simulink model "bike_model"  (R2018a)
settings: Solver=FixedStepAuto  StartTime=0.0  StopTime=10  FixedStep=Ts_IMU  RelTol=1e-3
values from neighbouring files (symbols this model uses):
  A_full = zeros(length(velocity_lqr),3,3)    [bike_init.m]
  A_full_dis = zeros(length(velocity_lqr),3,3)    [bike_init.m]
  amp_dist_roll_rate = 1    [bike_init.m]
  b = 1.095    [bike_init.m]    (also in bike_init_Merged_v1.m = bike3D190215())
  B_full = zeros(length(velocity_lqr),3)    [bike_init.m]
  B_full_dis = zeros(length(velocity_lqr),3)    [bike_init.m]
  C = eye(3)    [bike_init.m]    (also in bike_init_Merged_v1.m)
  complementary = 0.995    [bike_init.m]    (also in bike_init_Merged_v1.m = 0.985)
  cumulative_dist_along_path = [0;cumsum(dist_from_vertex_to_vertex,1)]    [bike_init.m]    (also in bike_init_Merged_v1.m)
  Dead_Band = [0.055,-0.005,0.005]    [bike_init.m]    (also in bike_init_Merged_v1.m = [0.055,-0.055,0.005])
  delay = 0.045    [bike_init.m]    (also in bike_init_Merged_v1.m)
  discrete = 1    [bike_init.m]
  dist_freq = 100    [bike_init.m]
  g = 9.81    [bike_init.m]    (also in bike_init_Merged_v1.m)
  IMU_height = 0.9    [bike_init.m]
  initial_x = x_ini_diff    (= 0)    [bike_init.m]    (also in bike_init_Merged_v1.m)
  initial_y = y_ini_diff    (= 0)    [bike_init.m]    (also in bike_init_Merged_v1.m)
  input_velocity = 2    [bike_init.m]    (also in bike_init_Merged_v1.m = 2.5)
  K_full = zeros(length(velocity_lqr),3)    [bike_init.m]
  K_full_dis = zeros(length(velocity_lqr),3)    [bike_init.m]    (also in bike_init_Merged_v1.m)
  L_full = zeros(length(velocity_lqr),3,3)    [bike_init.m]
  L_full_dis = zeros(length(velocity_lqr),3,3)    [bike_init.m]
  max_handlebar = 40*(pi/180)    (= 0.698131700798)    [bike_init.m]    (also in bike_init_Merged_v1.m)
  max_steering_motor_acc = inf    [bike_init.m]    (also in bike_init_Merged_v1.m)
  max_steering_motor_speed = 7.5    [bike_init.m]    (also in bike_init_Merged_v1.m)
  min_handlebar = -max_handlebar    (= -0.698131700798)    [bike_init.m]    (also in bike_init_Merged_v1.m)
  min_steering_motor_acc = -inf    [bike_init.m]    (also in bike_init_Merged_v1.m)
  min_steering_motor_speed = -7.5    [bike_init.m]    (also in bike_init_Merged_v1.m)
  noise_acc = 0.006*(pi/180)    (= 0.00010471975512)    [bike_init.m]    (also in bike_init_Merged_v1.m)
  noise_encoder = 1e-7    (= 1e-07)    [bike_init.m]    (also in bike_init_Merged_v1.m)
  noise_gyro = 0.001929307*(pi/180)    (= 3.36727594318e-05)    [bike_init.m]    (also in bike_init_Merged_v1.m)
  noise_hall = 0    [bike_init.m]    (also in bike_init_Merged_v1.m)
  parameters = [g h b a]    [bike_init.m]
  path_x = time_array    [bike_init.m]    (also in bike_init_Merged_v1.m)
  path_y = sqrt(path_x * 0.8) .* sin(0.1*path_x)    [bike_init.m]    (also in bike_init_Merged_v1.m)
  roll_rate_coef = 0.8    [bike_init.m]    (also in bike_init_Merged_v1.m = 0.9)
  Ts = 0.04    [bike_init.m]    (also in bike_init_Merged_v1.m)
  Ts_IMU = 0.01    [bike_init.m]    (also in bike_init_Merged_v1.m = 0.04)
  velocity_lqr = linspace(0.001,10,100)    [bike_init.m]    (also in bike_init_Merged_v1.m = [velocity_lqr-0.1 velocity_lqr velocity_lqr+0.1])
undefined symbols (not defined in the file or in its folder): curvature
libraries: simulink x14, dspsigops x2, dspsigattribs x1
(part 2 of 3)

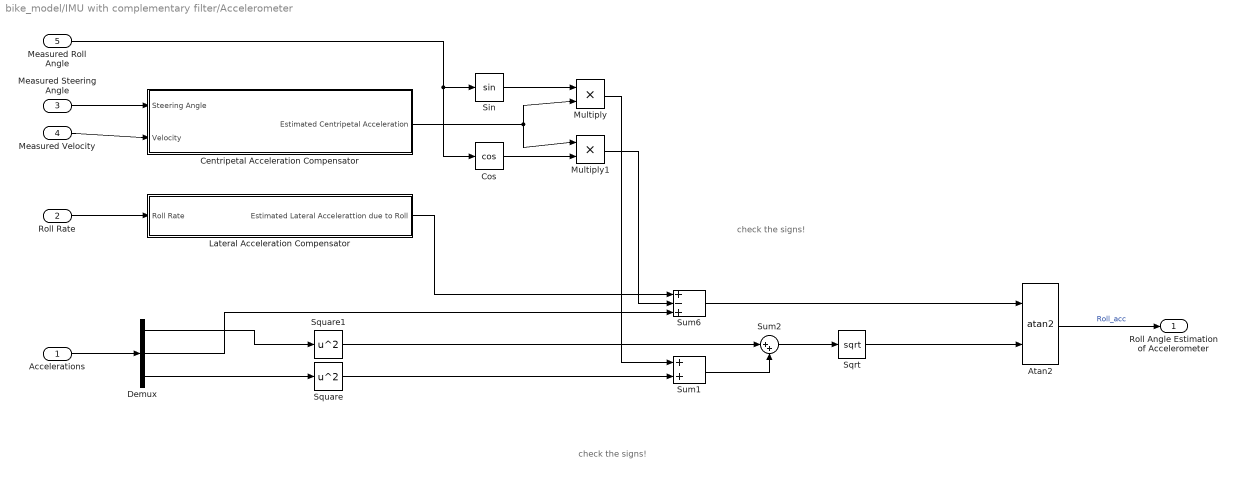
== system bike_model/IMU with complementary filter/Accelerometer ==
  note: check the signs!
  note: check the signs!
  Accelerations : Inport
  Roll Rate : Inport  Port=2
  Measured Steering Angle : Inport  Port=3
  Measured Velocity : Inport  Port=4
  Measured Roll Angle : Inport  Port=5
  Atan2 : Trigonometry  Operator=atan2
  Centripetal Acceleration Compensator : Subsystem
  Cos : Trigonometry  Operator=cos
  Demux : Demux  Outputs=3
  Lateral Acceleration Compensator : Subsystem
  Multiply : Product
  Multiply1 : Product
  Sin : Trigonometry
  Sqrt : Sqrt  SaturateOnIntegerOverflow=on
  Square : Math  Operator=square  SaturateOnIntegerOverflow=on
  Square1 : Math  Operator=square  SaturateOnIntegerOverflow=on
  Sum1 : Sum
  Sum2 : Sum  Inputs=|++
  Sum6 : Sum  Inputs=+-+
  Roll Angle Estimation of Accelerometer : Outport
  wires:
  Sum6/1 -> Atan2/1
  Sum2/1 -> Sqrt/1
  Square1/1 -> Sum2/1
  Demux/1 -> Square1/1
  Sum1/1 -> Sum2/2
  Sqrt/1 -> Atan2/2
  Lateral Acceleration Compensator/1(Estimated Lateral Accelerattion due to Roll) -> Sum6/1
  Atan2/1 -> Roll Angle Estimation of Accelerometer/1  "Roll_acc"
  Roll Rate/1 -> Lateral Acceleration Compensator/1(Roll Rate)
  Demux/3 -> Square/1
  Demux/2 -> Sum6/3
  Accelerations/1 -> Demux/1
  Measured Velocity/1 -> Centripetal Acceleration Compensator/2(Velocity)
  Measured Steering Angle/1 -> Centripetal Acceleration Compensator/1(Steering Angle)
  Centripetal Acceleration Compensator/1(Estimated Centripetal Acceleration) -> Multiply1/1, Multiply/2
  Measured Roll Angle/1 -> Sin/1, Cos/1
  Cos/1 -> Multiply1/2
  Sin/1 -> Multiply/1
  Multiply1/1 -> Sum6/2
  Square/1 -> Sum1/2
  Multiply/1 -> Sum1/1

== system bike_model/IMU with complementary filter/Complementary Filter ==
  Noise Enable : Inport
  Roll Angle Estimation due to Accelerometer : Inport  Port=2
  Roll Rate due to Gyroscope : Inport  Port=3
  Delay : Delay  DelayLength=1
  Gain2 : Gain  Gain=complementary
  Gain3 : Gain  Gain=1-complementary
  Gain4 : Gain  Gain=Ts_IMU
  Noise on accelerometer estimation : RandomNumber  Variance=noise_acc  Seed=3  SampleTime=Ts_IMU
  Sum3 : Sum  Inputs=|++
  Sum4 : Sum  Inputs=++|
  Sum5 : Sum  Inputs=++|
  Switch3 : Switch  Criteria=u2 > Threshold
  Roll Angle Estimation : Outport
  wires:
  Roll Angle Estimation due to Accelerometer/1 -> Sum5/2  "Roll_acc"
  Sum3/1 -> Gain2/1
  Sum5/1 -> Gain3/1
  Roll Rate due to Gyroscope/1 -> Gain4/1
  Switch3/1 -> Sum5/1
  Noise on accelerometer estimation/1 -> Switch3/1
  Delay/1 -> Sum3/2
  Gain4/1 -> Sum3/1
  Noise Enable/1 -> Switch3/2
  Gain2/1 -> Sum4/2
  Gain3/1 -> Sum4/1
  Sum4/1 -> Delay/1, Roll Angle Estimation/1

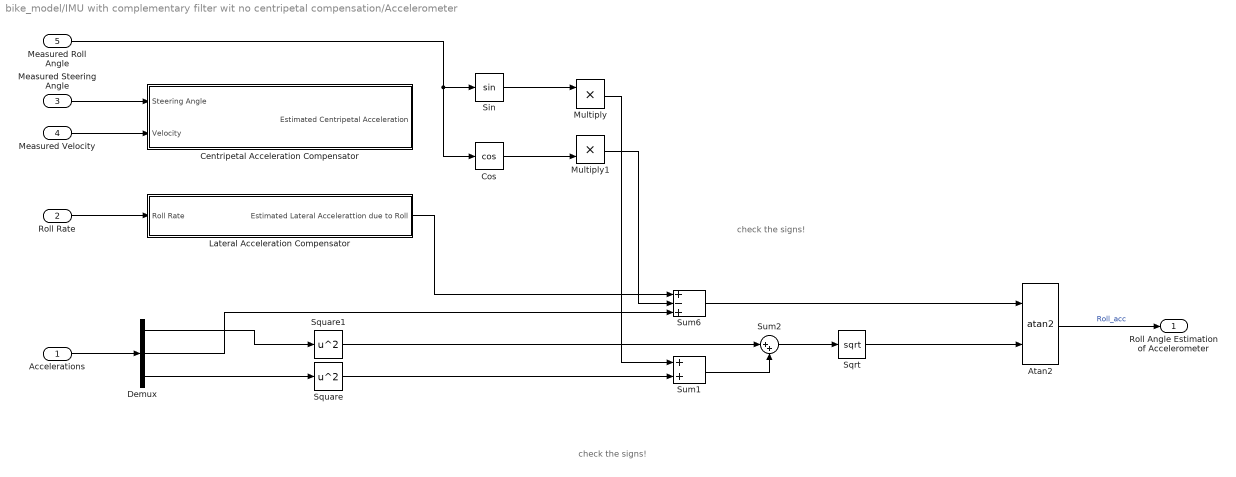
== system bike_model/IMU with complementary filter wit no centripetal compensation/Accelerometer ==
  note: check the signs!
  note: check the signs!
  Accelerations : Inport
  Roll Rate : Inport  Port=2
  Measured Steering Angle : Inport  Port=3
  Measured Velocity : Inport  Port=4
  Measured Roll Angle : Inport  Port=5
  Atan2 : Trigonometry  Operator=atan2
  Centripetal Acceleration Compensator : Subsystem
  Cos : Trigonometry  Operator=cos
  Demux : Demux  Outputs=3
  Lateral Acceleration Compensator : Subsystem
  Multiply : Product
  Multiply1 : Product
  Sin : Trigonometry
  Sqrt : Sqrt  SaturateOnIntegerOverflow=on
  Square : Math  Operator=square  SaturateOnIntegerOverflow=on
  Square1 : Math  Operator=square  SaturateOnIntegerOverflow=on
  Sum1 : Sum
  Sum2 : Sum  Inputs=|++
  Sum6 : Sum  Inputs=+-+
  Roll Angle Estimation of Accelerometer : Outport
  wires:
  Sum6/1 -> Atan2/1
  Sum2/1 -> Sqrt/1
  Square1/1 -> Sum2/1
  Demux/1 -> Square1/1
  Sum1/1 -> Sum2/2
  Sqrt/1 -> Atan2/2
  Lateral Acceleration Compensator/1(Estimated Lateral Accelerattion due to Roll) -> Sum6/1
  Atan2/1 -> Roll Angle Estimation of Accelerometer/1  "Roll_acc"
  Roll Rate/1 -> Lateral Acceleration Compensator/1(Roll Rate)
  Demux/3 -> Square/1
  Demux/2 -> Sum6/3
  Accelerations/1 -> Demux/1
  Measured Velocity/1 -> Centripetal Acceleration Compensator/2(Velocity)
  Measured Steering Angle/1 -> Centripetal Acceleration Compensator/1(Steering Angle)
  ? -> Multiply1/1, Multiply/2
  Measured Roll Angle/1 -> Sin/1, Cos/1
  Cos/1 -> Multiply1/2
  Sin/1 -> Multiply/1
  Multiply1/1 -> Sum6/2
  Square/1 -> Sum1/2
  Multiply/1 -> Sum1/1

== system bike_model/IMU with complementary filter wit no centripetal compensation/Complementary Filter ==
  Noise Enable : Inport
  Roll Angle Estimation due to Accelerometer : Inport  Port=2
  Roll Rate due to Gyroscope : Inport  Port=3
  Delay : Delay  DelayLength=1
  Gain2 : Gain  Gain=complementary
  Gain3 : Gain  Gain=1-complementary
  Gain4 : Gain  Gain=Ts_IMU
  Noise on accelerometer estimation : RandomNumber  Variance=noise_acc  Seed=3  SampleTime=Ts_IMU
  Sum3 : Sum  Inputs=|++
  Sum4 : Sum  Inputs=++|
  Sum5 : Sum  Inputs=++|
  Switch3 : Switch  Criteria=u2 > Threshold
  Roll Angle Estimation : Outport
  wires:
  Roll Angle Estimation due to Accelerometer/1 -> Sum5/2  "Roll_acc"
  Sum3/1 -> Gain2/1
  Sum5/1 -> Gain3/1
  Roll Rate due to Gyroscope/1 -> Gain4/1
  Switch3/1 -> Sum5/1
  Noise on accelerometer estimation/1 -> Switch3/1
  Delay/1 -> Sum3/2
  Gain4/1 -> Sum3/1
  Noise Enable/1 -> Switch3/2
  Gain2/1 -> Sum4/2
  Gain3/1 -> Sum4/1
  Sum4/1 -> Delay/1, Roll Angle Estimation/1

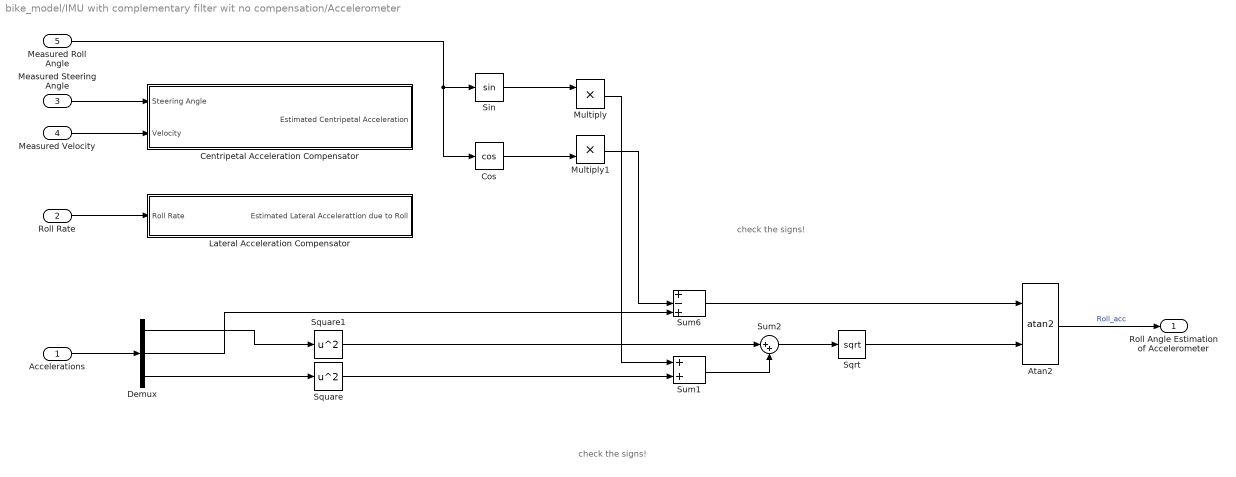
== system bike_model/IMU with complementary filter wit no compensation/Accelerometer ==
  note: check the signs!
  note: check the signs!
  Accelerations : Inport
  Roll Rate : Inport  Port=2
  Measured Steering Angle : Inport  Port=3
  Measured Velocity : Inport  Port=4
  Measured Roll Angle : Inport  Port=5
  Atan2 : Trigonometry  Operator=atan2
  Centripetal Acceleration Compensator : Subsystem
  Cos : Trigonometry  Operator=cos
  Demux : Demux  Outputs=3
  Lateral Acceleration Compensator : Subsystem
  Multiply : Product
  Multiply1 : Product
  Sin : Trigonometry
  Sqrt : Sqrt  SaturateOnIntegerOverflow=on
  Square : Math  Operator=square  SaturateOnIntegerOverflow=on
  Square1 : Math  Operator=square  SaturateOnIntegerOverflow=on
  Sum1 : Sum
  Sum2 : Sum  Inputs=|++
  Sum6 : Sum  Inputs=+-+
  Roll Angle Estimation of Accelerometer : Outport
  wires:
  Sum6/1 -> Atan2/1
  Sum2/1 -> Sqrt/1
  Square1/1 -> Sum2/1
  Demux/1 -> Square1/1
  Sum1/1 -> Sum2/2
  Sqrt/1 -> Atan2/2
  ? -> Sum6/1
  Atan2/1 -> Roll Angle Estimation of Accelerometer/1  "Roll_acc"
  Roll Rate/1 -> Lateral Acceleration Compensator/1(Roll Rate)
  Demux/3 -> Square/1
  Demux/2 -> Sum6/3
  Accelerations/1 -> Demux/1
  Measured Velocity/1 -> Centripetal Acceleration Compensator/2(Velocity)
  Measured Steering Angle/1 -> Centripetal Acceleration Compensator/1(Steering Angle)
  ? -> Multiply1/1, Multiply/2
  Measured Roll Angle/1 -> Sin/1, Cos/1
  Cos/1 -> Multiply1/2
  Sin/1 -> Multiply/1
  Multiply1/1 -> Sum6/2
  Square/1 -> Sum1/2
  Multiply/1 -> Sum1/1

== system bike_model/IMU with complementary filter wit no compensation/Complementary Filter ==
  Noise Enable : Inport
  Roll Angle Estimation due to Accelerometer : Inport  Port=2
  Roll Rate due to Gyroscope : Inport  Port=3
  Delay : Delay  DelayLength=1
  Gain2 : Gain  Gain=complementary
  Gain3 : Gain  Gain=1-complementary
  Gain4 : Gain  Gain=Ts_IMU
  Noise on accelerometer estimation : RandomNumber  Variance=noise_acc  Seed=3  SampleTime=Ts_IMU
  Sum3 : Sum  Inputs=|++
  Sum4 : Sum  Inputs=++|
  Sum5 : Sum  Inputs=++|
  Switch3 : Switch  Criteria=u2 > Threshold
  Roll Angle Estimation : Outport
  wires:
  Roll Angle Estimation due to Accelerometer/1 -> Sum5/2  "Roll_acc"
  Sum3/1 -> Gain2/1
  Sum5/1 -> Gain3/1
  Roll Rate due to Gyroscope/1 -> Gain4/1
  Switch3/1 -> Sum5/1
  Noise on accelerometer estimation/1 -> Switch3/1
  Delay/1 -> Sum3/2
  Gain4/1 -> Sum3/1
  Noise Enable/1 -> Switch3/2
  Gain2/1 -> Sum4/2
  Gain3/1 -> Sum4/1
  Sum4/1 -> Delay/1, Roll Angle Estimation/1

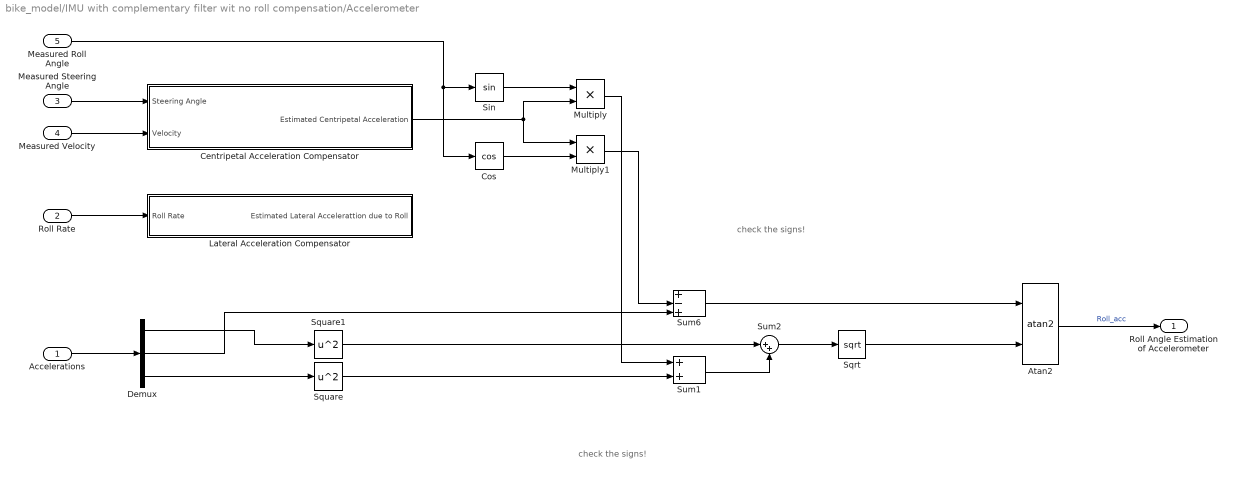
== system bike_model/IMU with complementary filter wit no roll compensation/Accelerometer ==
  note: check the signs!
  note: check the signs!
  Accelerations : Inport
  Roll Rate : Inport  Port=2
  Measured Steering Angle : Inport  Port=3
  Measured Velocity : Inport  Port=4
  Measured Roll Angle : Inport  Port=5
  Atan2 : Trigonometry  Operator=atan2
  Centripetal Acceleration Compensator : Subsystem
  Cos : Trigonometry  Operator=cos
  Demux : Demux  Outputs=3
  Lateral Acceleration Compensator : Subsystem
  Multiply : Product
  Multiply1 : Product
  Sin : Trigonometry
  Sqrt : Sqrt  SaturateOnIntegerOverflow=on
  Square : Math  Operator=square  SaturateOnIntegerOverflow=on
  Square1 : Math  Operator=square  SaturateOnIntegerOverflow=on
  Sum1 : Sum
  Sum2 : Sum  Inputs=|++
  Sum6 : Sum  Inputs=+-+
  Roll Angle Estimation of Accelerometer : Outport
  wires:
  Sum6/1 -> Atan2/1
  Sum2/1 -> Sqrt/1
  Square1/1 -> Sum2/1
  Demux/1 -> Square1/1
  Sum1/1 -> Sum2/2
  Sqrt/1 -> Atan2/2
  ? -> Sum6/1
  Atan2/1 -> Roll Angle Estimation of Accelerometer/1  "Roll_acc"
  Roll Rate/1 -> Lateral Acceleration Compensator/1(Roll Rate)
  Demux/3 -> Square/1
  Demux/2 -> Sum6/3
  Accelerations/1 -> Demux/1
  Measured Velocity/1 -> Centripetal Acceleration Compensator/2(Velocity)
  Measured Steering Angle/1 -> Centripetal Acceleration Compensator/1(Steering Angle)
  Centripetal Acceleration Compensator/1(Estimated Centripetal Acceleration) -> Multiply1/1, Multiply/2
  Measured Roll Angle/1 -> Sin/1, Cos/1
  Cos/1 -> Multiply1/2
  Sin/1 -> Multiply/1
  Multiply1/1 -> Sum6/2
  Square/1 -> Sum1/2
  Multiply/1 -> Sum1/1

== system bike_model/IMU with complementary filter wit no roll compensation/Complementary Filter ==
  Noise Enable : Inport
  Roll Angle Estimation due to Accelerometer : Inport  Port=2
  Roll Rate due to Gyroscope : Inport  Port=3
  Delay : Delay  DelayLength=1
  Gain2 : Gain  Gain=complementary
  Gain3 : Gain  Gain=1-complementary
  Gain4 : Gain  Gain=Ts_IMU
  Noise on accelerometer estimation : RandomNumber  Variance=noise_acc  Seed=3  SampleTime=Ts_IMU
  Sum3 : Sum  Inputs=|++
  Sum4 : Sum  Inputs=++|
  Sum5 : Sum  Inputs=++|
  Switch3 : Switch  Criteria=u2 > Threshold
  Roll Angle Estimation : Outport
  wires:
  Roll Angle Estimation due to Accelerometer/1 -> Sum5/2  "Roll_acc"
  Sum3/1 -> Gain2/1
  Sum5/1 -> Gain3/1
  Roll Rate due to Gyroscope/1 -> Gain4/1
  Switch3/1 -> Sum5/1
  Noise on accelerometer estimation/1 -> Switch3/1
  Delay/1 -> Sum3/2
  Gain4/1 -> Sum3/1
  Noise Enable/1 -> Switch3/2
  Gain2/1 -> Sum4/2
  Gain3/1 -> Sum4/1
  Sum4/1 -> Delay/1, Roll Angle Estimation/1

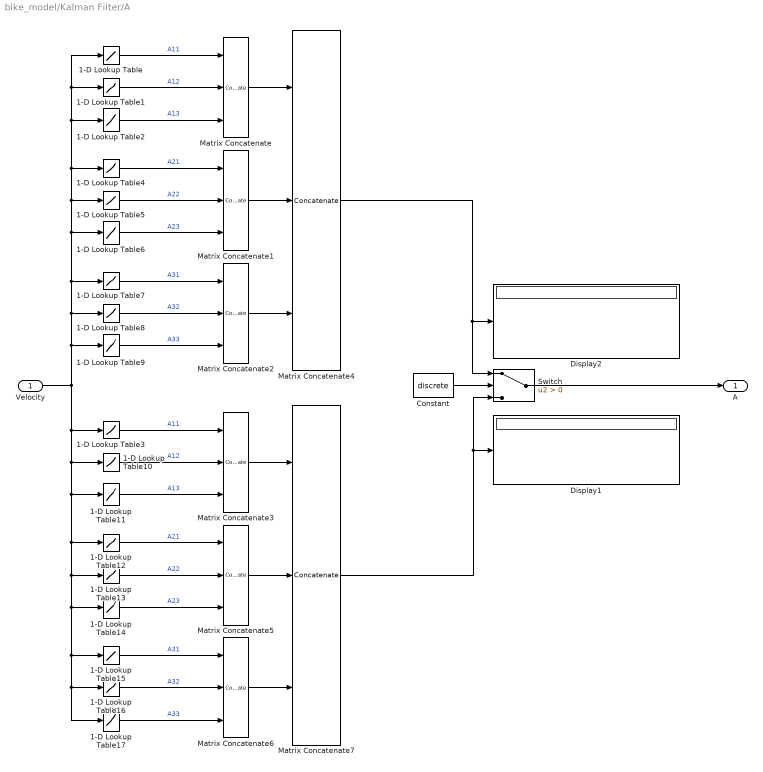
== system bike_model/Kalman Filter/A ==
  Velocity : Inport
  1-D Lookup Table : Lookup_n-D  NumberOfTableDimensions=1  BreakpointsForDimension1=velocity_lqr  BreakpointsForDimension2=velocity_lqr  BreakpointsForDimension3=velocity_lqr  BreakpointsForDimension4=velocity_lqr  Table=A_full_dis(:,1,1)  InternalRulePriority=Speed  RndMeth=Simplest  InputSameDT=on
  1-D Lookup Table1 : Lookup_n-D  NumberOfTableDimensions=1  BreakpointsForDimension1=velocity_lqr  BreakpointsForDimension2=velocity_lqr  BreakpointsForDimension3=velocity_lqr  BreakpointsForDimension4=velocity_lqr  Table=A_full_dis(:,1,2)  InternalRulePriority=Speed  RndMeth=Simplest  InputSameDT=on
  1-D Lookup Table10 : Lookup_n-D  NumberOfTableDimensions=1  BreakpointsForDimension1=velocity_lqr  BreakpointsForDimension2=velocity_lqr  BreakpointsForDimension3=velocity_lqr  BreakpointsForDimension4=velocity_lqr  Table=A_full(:,1,2)  InternalRulePriority=Speed  RndMeth=Simplest  InputSameDT=on
  1-D Lookup Table11 : Lookup_n-D  NumberOfTableDimensions=1  BreakpointsForDimension1=velocity_lqr  BreakpointsForDimension2=velocity_lqr  BreakpointsForDimension3=velocity_lqr  BreakpointsForDimension4=velocity_lqr  Table=A_full(:,1,3)  InternalRulePriority=Speed  RndMeth=Simplest  InputSameDT=on
  1-D Lookup Table12 : Lookup_n-D  NumberOfTableDimensions=1  BreakpointsForDimension1=velocity_lqr  BreakpointsForDimension2=velocity_lqr  BreakpointsForDimension3=velocity_lqr  BreakpointsForDimension4=velocity_lqr  Table=A_full(:,2,1)  InternalRulePriority=Speed  RndMeth=Simplest  InputSameDT=on
  1-D Lookup Table13 : Lookup_n-D  NumberOfTableDimensions=1  BreakpointsForDimension1=velocity_lqr  BreakpointsForDimension2=velocity_lqr  BreakpointsForDimension3=velocity_lqr  BreakpointsForDimension4=velocity_lqr  Table=A_full(:,2,2)  InternalRulePriority=Speed  RndMeth=Simplest  InputSameDT=on
  1-D Lookup Table14 : Lookup_n-D  NumberOfTableDimensions=1  BreakpointsForDimension1=velocity_lqr  BreakpointsForDimension2=velocity_lqr  BreakpointsForDimension3=velocity_lqr  BreakpointsForDimension4=velocity_lqr  Table=A_full(:,2,3)  InternalRulePriority=Speed  RndMeth=Simplest  InputSameDT=on
  1-D Lookup Table15 : Lookup_n-D  NumberOfTableDimensions=1  BreakpointsForDimension1=velocity_lqr  BreakpointsForDimension2=velocity_lqr  BreakpointsForDimension3=velocity_lqr  BreakpointsForDimension4=velocity_lqr  Table=A_full(:,3,1)  InternalRulePriority=Speed  RndMeth=Simplest  InputSameDT=on
  1-D Lookup Table16 : Lookup_n-D  NumberOfTableDimensions=1  BreakpointsForDimension1=velocity_lqr  BreakpointsForDimension2=velocity_lqr  BreakpointsForDimension3=velocity_lqr  BreakpointsForDimension4=velocity_lqr  Table=A_full(:,3,2)  InternalRulePriority=Speed  RndMeth=Simplest  InputSameDT=on
  1-D Lookup Table17 : Lookup_n-D  NumberOfTableDimensions=1  BreakpointsForDimension1=velocity_lqr  BreakpointsForDimension2=velocity_lqr  BreakpointsForDimension3=velocity_lqr  BreakpointsForDimension4=velocity_lqr  Table=A_full(:,3,3)  InternalRulePriority=Speed  RndMeth=Simplest  InputSameDT=on
  1-D Lookup Table2 : Lookup_n-D  NumberOfTableDimensions=1  BreakpointsForDimension1=velocity_lqr  BreakpointsForDimension2=velocity_lqr  BreakpointsForDimension3=velocity_lqr  BreakpointsForDimension4=velocity_lqr  Table=A_full_dis(:,1,3)  InternalRulePriority=Speed  RndMeth=Simplest  InputSameDT=on
  1-D Lookup Table3 : Lookup_n-D  NumberOfTableDimensions=1  BreakpointsForDimension1=velocity_lqr  BreakpointsForDimension2=velocity_lqr  BreakpointsForDimension3=velocity_lqr  BreakpointsForDimension4=velocity_lqr  Table=A_full(:,1,1)  InternalRulePriority=Speed  RndMeth=Simplest  InputSameDT=on
  1-D Lookup Table4 : Lookup_n-D  NumberOfTableDimensions=1  BreakpointsForDimension1=velocity_lqr  BreakpointsForDimension2=velocity_lqr  BreakpointsForDimension3=velocity_lqr  BreakpointsForDimension4=velocity_lqr  Table=A_full_dis(:,2,1)  InternalRulePriority=Speed  RndMeth=Simplest  InputSameDT=on
  1-D Lookup Table5 : Lookup_n-D  NumberOfTableDimensions=1  BreakpointsForDimension1=velocity_lqr  BreakpointsForDimension2=velocity_lqr  BreakpointsForDimension3=velocity_lqr  BreakpointsForDimension4=velocity_lqr  Table=A_full_dis(:,2,2)  InternalRulePriority=Speed  RndMeth=Simplest  InputSameDT=on
  1-D Lookup Table6 : Lookup_n-D  NumberOfTableDimensions=1  BreakpointsForDimension1=velocity_lqr  BreakpointsForDimension2=velocity_lqr  BreakpointsForDimension3=velocity_lqr  BreakpointsForDimension4=velocity_lqr  Table=A_full_dis(:,2,3)  InternalRulePriority=Speed  RndMeth=Simplest  InputSameDT=on
  1-D Lookup Table7 : Lookup_n-D  NumberOfTableDimensions=1  BreakpointsForDimension1=velocity_lqr  BreakpointsForDimension2=velocity_lqr  BreakpointsForDimension3=velocity_lqr  BreakpointsForDimension4=velocity_lqr  Table=A_full_dis(:,3,1)  InternalRulePriority=Speed  RndMeth=Simplest  InputSameDT=on
  1-D Lookup Table8 : Lookup_n-D  NumberOfTableDimensions=1  BreakpointsForDimension1=velocity_lqr  BreakpointsForDimension2=velocity_lqr  BreakpointsForDimension3=velocity_lqr  BreakpointsForDimension4=velocity_lqr  Table=A_full_dis(:,3,2)  InternalRulePriority=Speed  RndMeth=Simplest  InputSameDT=on
  1-D Lookup Table9 : Lookup_n-D  NumberOfTableDimensions=1  BreakpointsForDimension1=velocity_lqr  BreakpointsForDimension2=velocity_lqr  BreakpointsForDimension3=velocity_lqr  BreakpointsForDimension4=velocity_lqr  Table=A_full_dis(:,3,3)  InternalRulePriority=Speed  RndMeth=Simplest  InputSameDT=on
  Constant : Constant  Value=discrete
  Display1 : Display
  Display2 : Display
  Matrix Concatenate{,1..3,5..6} (6 alike) : Concatenate  NumInputs=3  Mode=Multidimensional array  ConcatenateDimension=2
  Matrix Concatenate4 : Concatenate  NumInputs=3  Mode=Multidimensional array
  Matrix Concatenate7 : Concatenate  NumInputs=3  Mode=Multidimensional array
  Switch : Switch  Criteria=u2 > Threshold
  A : Outport
  wires:
  1-D Lookup Table/1 -> Matrix Concatenate/1  "A11"
  1-D Lookup Table1/1 -> Matrix Concatenate/2  "A12"
  1-D Lookup Table2/1 -> Matrix Concatenate/3  "A13"
  1-D Lookup Table6/1 -> Matrix Concatenate1/3  "A23"
  1-D Lookup Table5/1 -> Matrix Concatenate1/2  "A22"
  1-D Lookup Table4/1 -> Matrix Concatenate1/1  "A21"
  1-D Lookup Table9/1 -> Matrix Concatenate2/3  "A33"
  1-D Lookup Table8/1 -> Matrix Concatenate2/2  "A32"
  1-D Lookup Table7/1 -> Matrix Concatenate2/1  "A31"
  Matrix Concatenate/1 -> Matrix Concatenate4/1
  Matrix Concatenate1/1 -> Matrix Concatenate4/2
  Matrix Concatenate2/1 -> Matrix Concatenate4/3
  1-D Lookup Table13/1 -> Matrix Concatenate5/2  "A22"
  Matrix Concatenate5/1 -> Matrix Concatenate7/2
  1-D Lookup Table11/1 -> Matrix Concatenate3/3  "A13"
  Matrix Concatenate6/1 -> Matrix Concatenate7/3
  1-D Lookup Table15/1 -> Matrix Concatenate6/1  "A31"
  Velocity/1 -> 1-D Lookup Table/1, 1-D Lookup Table1/1, 1-D Lookup Table2/1, 1-D Lookup Table4/1, 1-D Lookup Table5/1, 1-D Lookup Table6/1, 1-D Lookup Table7/1, 1-D Lookup Table8/1, 1-D Lookup Table9/1, 1-D Lookup Table17/1, 1-D Lookup Table16/1, 1-D Lookup Table15/1, 1-D Lookup Table14/1, 1-D Lookup Table13/1, 1-D Lookup Table12/1, 1-D Lookup Table11/1, 1-D Lookup Table10/1, 1-D Lookup Table3/1
  1-D Lookup Table14/1 -> Matrix Concatenate5/3  "A23"
  1-D Lookup Table12/1 -> Matrix Concatenate5/1  "A21"
  1-D Lookup Table3/1 -> Matrix Concatenate3/1  "A11"
  1-D Lookup Table16/1 -> Matrix Concatenate6/2  "A32"
  Matrix Concatenate3/1 -> Matrix Concatenate7/1
  1-D Lookup Table10/1 -> Matrix Concatenate3/2  "A12"
  1-D Lookup Table17/1 -> Matrix Concatenate6/3  "A33"
  Matrix Concatenate7/1 -> Display1/1, Switch/3
  Switch/1 -> A/1
  Constant/1 -> Switch/2
  Matrix Concatenate4/1 -> Display2/1, Switch/1

== system bike_model/Kalman Filter/B ==
  Velocity : Inport
  1-D Lookup Table : Lookup_n-D  NumberOfTableDimensions=1  BreakpointsForDimension1=velocity_lqr  BreakpointsForDimension2=velocity_lqr  BreakpointsForDimension3=velocity_lqr  BreakpointsForDimension4=velocity_lqr  Table=B_full_dis(:,1)  InternalRulePriority=Speed  RndMeth=Simplest  InputSameDT=on
  1-D Lookup Table1 : Lookup_n-D  NumberOfTableDimensions=1  BreakpointsForDimension1=velocity_lqr  BreakpointsForDimension2=velocity_lqr  BreakpointsForDimension3=velocity_lqr  BreakpointsForDimension4=velocity_lqr  Table=B_full_dis(:,2)  InternalRulePriority=Speed  RndMeth=Simplest  InputSameDT=on
  1-D Lookup Table10 : Lookup_n-D  NumberOfTableDimensions=1  BreakpointsForDimension1=velocity_lqr  BreakpointsForDimension2=velocity_lqr  BreakpointsForDimension3=velocity_lqr  BreakpointsForDimension4=velocity_lqr  Table=B_full(:,2)  InternalRulePriority=Speed  RndMeth=Simplest  InputSameDT=on
  1-D Lookup Table11 : Lookup_n-D  NumberOfTableDimensions=1  BreakpointsForDimension1=velocity_lqr  BreakpointsForDimension2=velocity_lqr  BreakpointsForDimension3=velocity_lqr  BreakpointsForDimension4=velocity_lqr  Table=B_full(:,3)  InternalRulePriority=Speed  RndMeth=Simplest  InputSameDT=on
  1-D Lookup Table2 : Lookup_n-D  NumberOfTableDimensions=1  BreakpointsForDimension1=velocity_lqr  BreakpointsForDimension2=velocity_lqr  BreakpointsForDimension3=velocity_lqr  BreakpointsForDimension4=velocity_lqr  Table=B_full_dis(:,3)  InternalRulePriority=Speed  RndMeth=Simplest  InputSameDT=on
  1-D Lookup Table3 : Lookup_n-D  NumberOfTableDimensions=1  BreakpointsForDimension1=velocity_lqr  BreakpointsForDimension2=velocity_lqr  BreakpointsForDimension3=velocity_lqr  BreakpointsForDimension4=velocity_lqr  Table=B_full(:,1)  InternalRulePriority=Speed  RndMeth=Simplest  InputSameDT=on
  Constant : Constant  Value=discrete
  Display1 : Display
  Display2 : Display
  Matrix Concatenate : Concatenate  NumInputs=3  Mode=Multidimensional array
  Matrix Concatenate3 : Concatenate  NumInputs=3  Mode=Multidimensional array
  Switch : Switch  Criteria=u2 > Threshold
  B : Outport
  wires:
  1-D Lookup Table/1 -> Matrix Concatenate/1  "B1"
  1-D Lookup Table1/1 -> Matrix Concatenate/2  "B2"
  1-D Lookup Table2/1 -> Matrix Concatenate/3  "B3"
  1-D Lookup Table11/1 -> Matrix Concatenate3/3  "B3"
  Velocity/1 -> 1-D Lookup Table/1, 1-D Lookup Table1/1, 1-D Lookup Table2/1, 1-D Lookup Table11/1, 1-D Lookup Table10/1, 1-D Lookup Table3/1
  1-D Lookup Table3/1 -> Matrix Concatenate3/1  "B1"
  1-D Lookup Table10/1 -> Matrix Concatenate3/2  "B2"
  Matrix Concatenate3/1 -> Display1/1, Switch/3
  Switch/1 -> B/1
  Constant/1 -> Switch/2
  Matrix Concatenate/1 -> Display2/1, Switch/1

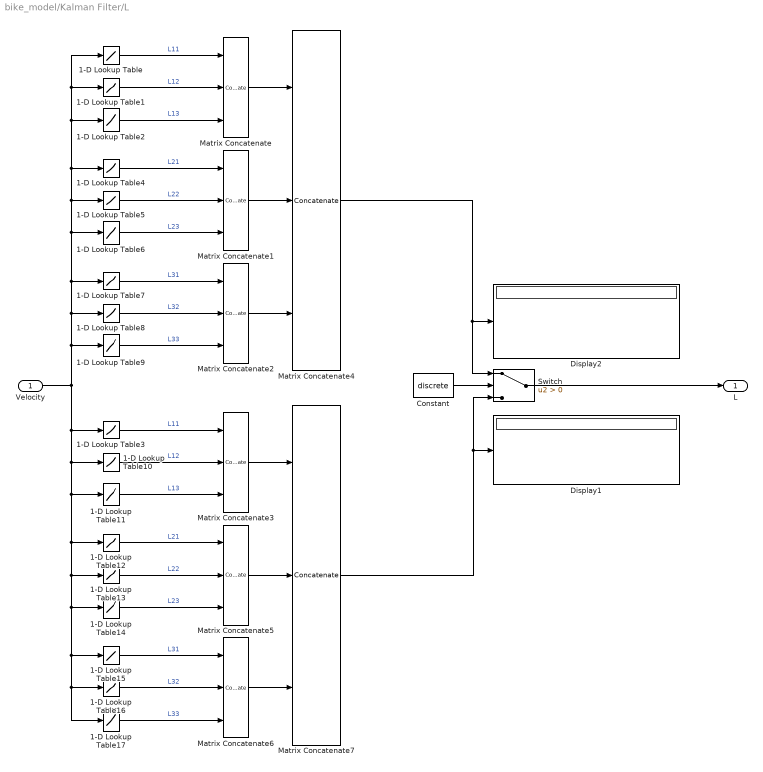
== system bike_model/Kalman Filter/L ==
  Velocity : Inport
  1-D Lookup Table : Lookup_n-D  NumberOfTableDimensions=1  BreakpointsForDimension1=velocity_lqr  BreakpointsForDimension2=velocity_lqr  BreakpointsForDimension3=velocity_lqr  BreakpointsForDimension4=velocity_lqr  Table=L_full_dis(:,1,1)  InternalRulePriority=Speed  RndMeth=Simplest  InputSameDT=on
  1-D Lookup Table1 : Lookup_n-D  NumberOfTableDimensions=1  BreakpointsForDimension1=velocity_lqr  BreakpointsForDimension2=velocity_lqr  BreakpointsForDimension3=velocity_lqr  BreakpointsForDimension4=velocity_lqr  Table=L_full_dis(:,1,2)  InternalRulePriority=Speed  RndMeth=Simplest  InputSameDT=on
  1-D Lookup Table10 : Lookup_n-D  NumberOfTableDimensions=1  BreakpointsForDimension1=velocity_lqr  BreakpointsForDimension2=velocity_lqr  BreakpointsForDimension3=velocity_lqr  BreakpointsForDimension4=velocity_lqr  Table=L_full(:,1,2)  InternalRulePriority=Speed  RndMeth=Simplest  InputSameDT=on
  1-D Lookup Table11 : Lookup_n-D  NumberOfTableDimensions=1  BreakpointsForDimension1=velocity_lqr  BreakpointsForDimension2=velocity_lqr  BreakpointsForDimension3=velocity_lqr  BreakpointsForDimension4=velocity_lqr  Table=L_full(:,1,3)  InternalRulePriority=Speed  RndMeth=Simplest  InputSameDT=on
  1-D Lookup Table12 : Lookup_n-D  NumberOfTableDimensions=1  BreakpointsForDimension1=velocity_lqr  BreakpointsForDimension2=velocity_lqr  BreakpointsForDimension3=velocity_lqr  BreakpointsForDimension4=velocity_lqr  Table=L_full(:,2,1)  InternalRulePriority=Speed  RndMeth=Simplest  InputSameDT=on
  1-D Lookup Table13 : Lookup_n-D  NumberOfTableDimensions=1  BreakpointsForDimension1=velocity_lqr  BreakpointsForDimension2=velocity_lqr  BreakpointsForDimension3=velocity_lqr  BreakpointsForDimension4=velocity_lqr  Table=L_full(:,2,2)  InternalRulePriority=Speed  RndMeth=Simplest  InputSameDT=on
  1-D Lookup Table14 : Lookup_n-D  NumberOfTableDimensions=1  BreakpointsForDimension1=velocity_lqr  BreakpointsForDimension2=velocity_lqr  BreakpointsForDimension3=velocity_lqr  BreakpointsForDimension4=velocity_lqr  Table=L_full(:,2,3)  InternalRulePriority=Speed  RndMeth=Simplest  InputSameDT=on
  1-D Lookup Table15 : Lookup_n-D  NumberOfTableDimensions=1  BreakpointsForDimension1=velocity_lqr  BreakpointsForDimension2=velocity_lqr  BreakpointsForDimension3=velocity_lqr  BreakpointsForDimension4=velocity_lqr  Table=L_full(:,3,1)  InternalRulePriority=Speed  RndMeth=Simplest  InputSameDT=on
  1-D Lookup Table16 : Lookup_n-D  NumberOfTableDimensions=1  BreakpointsForDimension1=velocity_lqr  BreakpointsForDimension2=velocity_lqr  BreakpointsForDimension3=velocity_lqr  BreakpointsForDimension4=velocity_lqr  Table=L_full(:,3,2)  InternalRulePriority=Speed  RndMeth=Simplest  InputSameDT=on
  1-D Lookup Table17 : Lookup_n-D  NumberOfTableDimensions=1  BreakpointsForDimension1=velocity_lqr  BreakpointsForDimension2=velocity_lqr  BreakpointsForDimension3=velocity_lqr  BreakpointsForDimension4=velocity_lqr  Table=L_full(:,3,3)  InternalRulePriority=Speed  RndMeth=Simplest  InputSameDT=on
  1-D Lookup Table2 : Lookup_n-D  NumberOfTableDimensions=1  BreakpointsForDimension1=velocity_lqr  BreakpointsForDimension2=velocity_lqr  BreakpointsForDimension3=velocity_lqr  BreakpointsForDimension4=velocity_lqr  Table=L_full_dis(:,1,3)  InternalRulePriority=Speed  RndMeth=Simplest  InputSameDT=on
  1-D Lookup Table3 : Lookup_n-D  NumberOfTableDimensions=1  BreakpointsForDimension1=velocity_lqr  BreakpointsForDimension2=velocity_lqr  BreakpointsForDimension3=velocity_lqr  BreakpointsForDimension4=velocity_lqr  Table=L_full(:,1,1)  InternalRulePriority=Speed  RndMeth=Simplest  InputSameDT=on
  1-D Lookup Table4 : Lookup_n-D  NumberOfTableDimensions=1  BreakpointsForDimension1=velocity_lqr  BreakpointsForDimension2=velocity_lqr  BreakpointsForDimension3=velocity_lqr  BreakpointsForDimension4=velocity_lqr  Table=L_full_dis(:,2,1)  InternalRulePriority=Speed  RndMeth=Simplest  InputSameDT=on
  1-D Lookup Table5 : Lookup_n-D  NumberOfTableDimensions=1  BreakpointsForDimension1=velocity_lqr  BreakpointsForDimension2=velocity_lqr  BreakpointsForDimension3=velocity_lqr  BreakpointsForDimension4=velocity_lqr  Table=L_full_dis(:,2,2)  InternalRulePriority=Speed  RndMeth=Simplest  InputSameDT=on
  1-D Lookup Table6 : Lookup_n-D  NumberOfTableDimensions=1  BreakpointsForDimension1=velocity_lqr  BreakpointsForDimension2=velocity_lqr  BreakpointsForDimension3=velocity_lqr  BreakpointsForDimension4=velocity_lqr  Table=L_full_dis(:,2,3)  InternalRulePriority=Speed  RndMeth=Simplest  InputSameDT=on
  1-D Lookup Table7 : Lookup_n-D  NumberOfTableDimensions=1  BreakpointsForDimension1=velocity_lqr  BreakpointsForDimension2=velocity_lqr  BreakpointsForDimension3=velocity_lqr  BreakpointsForDimension4=velocity_lqr  Table=L_full_dis(:,3,1)  InternalRulePriority=Speed  RndMeth=Simplest  InputSameDT=on
  1-D Lookup Table8 : Lookup_n-D  NumberOfTableDimensions=1  BreakpointsForDimension1=velocity_lqr  BreakpointsForDimension2=velocity_lqr  BreakpointsForDimension3=velocity_lqr  BreakpointsForDimension4=velocity_lqr  Table=L_full_dis(:,3,2)  InternalRulePriority=Speed  RndMeth=Simplest  InputSameDT=on
  1-D Lookup Table9 : Lookup_n-D  NumberOfTableDimensions=1  BreakpointsForDimension1=velocity_lqr  BreakpointsForDimension2=velocity_lqr  BreakpointsForDimension3=velocity_lqr  BreakpointsForDimension4=velocity_lqr  Table=L_full_dis(:,3,3)  InternalRulePriority=Speed  RndMeth=Simplest  InputSameDT=on
  Constant : Constant  Value=discrete
  Display1 : Display
  Display2 : Display
  Matrix Concatenate{,1..3,5..6} (6 alike) : Concatenate  NumInputs=3  Mode=Multidimensional array  ConcatenateDimension=2
  Matrix Concatenate4 : Concatenate  NumInputs=3  Mode=Multidimensional array
  Matrix Concatenate7 : Concatenate  NumInputs=3  Mode=Multidimensional array
  Switch : Switch  Criteria=u2 > Threshold
  L : Outport
  wires:
  1-D Lookup Table/1 -> Matrix Concatenate/1  "L11"
  1-D Lookup Table1/1 -> Matrix Concatenate/2  "L12"
  1-D Lookup Table2/1 -> Matrix Concatenate/3  "L13"
  1-D Lookup Table6/1 -> Matrix Concatenate1/3  "L23"
  1-D Lookup Table5/1 -> Matrix Concatenate1/2  "L22"
  1-D Lookup Table4/1 -> Matrix Concatenate1/1  "L21"
  1-D Lookup Table9/1 -> Matrix Concatenate2/3  "L33"
  1-D Lookup Table8/1 -> Matrix Concatenate2/2  "L32"
  1-D Lookup Table7/1 -> Matrix Concatenate2/1  "L31"
  Matrix Concatenate/1 -> Matrix Concatenate4/1
  Matrix Concatenate1/1 -> Matrix Concatenate4/2
  Matrix Concatenate2/1 -> Matrix Concatenate4/3
  1-D Lookup Table13/1 -> Matrix Concatenate5/2  "L22"
  Matrix Concatenate5/1 -> Matrix Concatenate7/2
  1-D Lookup Table11/1 -> Matrix Concatenate3/3  "L13"
  Matrix Concatenate6/1 -> Matrix Concatenate7/3
  1-D Lookup Table15/1 -> Matrix Concatenate6/1  "L31"
  Velocity/1 -> 1-D Lookup Table/1, 1-D Lookup Table1/1, 1-D Lookup Table2/1, 1-D Lookup Table4/1, 1-D Lookup Table5/1, 1-D Lookup Table6/1, 1-D Lookup Table7/1, 1-D Lookup Table8/1, 1-D Lookup Table9/1, 1-D Lookup Table17/1, 1-D Lookup Table16/1, 1-D Lookup Table15/1, 1-D Lookup Table14/1, 1-D Lookup Table13/1, 1-D Lookup Table12/1, 1-D Lookup Table11/1, 1-D Lookup Table10/1, 1-D Lookup Table3/1
  1-D Lookup Table14/1 -> Matrix Concatenate5/3  "L23"
  1-D Lookup Table12/1 -> Matrix Concatenate5/1  "L21"
  1-D Lookup Table3/1 -> Matrix Concatenate3/1  "L11"
  1-D Lookup Table16/1 -> Matrix Concatenate6/2  "L32"
  Matrix Concatenate3/1 -> Matrix Concatenate7/1
  1-D Lookup Table10/1 -> Matrix Concatenate3/2  "L12"
  1-D Lookup Table17/1 -> Matrix Concatenate6/3  "L33"
  Matrix Concatenate7/1 -> Display1/1, Switch/3
  Switch/1 -> L/1
  Constant/1 -> Switch/2
  Matrix Concatenate4/1 -> Display2/1, Switch/1

== system bike_model/Maxon Motor/Motor Deadband ==
  Calculated Input : Inport
  Abs : Abs
  Abs1 : Abs
  Constant : Constant  Value=0  SampleTime=Ts
  Constant1 : Constant  Value=0  SampleTime=Ts
  Constant2 : Constant  Value=Dead_Band(2)  SampleTime=Ts
  Constant4 : Constant  Value=Dead_Band(1)  SampleTime=Ts
  Gain : Gain  Gain=-1
  Relay1 : Relay  OnSwitchValue=Dead_Band(3)  OffSwitchValue=-Dead_Band(3)
  Relay2 : Relay  OnSwitchValue=Dead_Band(3)  OffSwitchValue=-Dead_Band(3)
  Sum1 : Sum  Inputs=-+|
  Sum2 : Sum  Inputs=-+|
  Switch : Switch  Criteria=u2 > Threshold
  Switch1 : Switch  Criteria=u2 > Threshold
  Switch2 : Switch  Criteria=u2 > Threshold
  Input Signal After Dead Band : Outport
  wires:
  Constant4/1 -> Sum1/1
  Sum1/1 -> Relay1/1
  Relay1/1 -> Switch/2
  Switch/1 -> Switch1/1
  Constant/1 -> Switch/3
  Switch1/1 -> Input Signal After Dead Band/1
  Switch2/1 -> Switch1/3
  Constant1/1 -> Switch2/3
  Gain/1 -> Sum2/1
  Calculated Input/1 -> Abs/1, Switch2/1, Abs1/1, Switch/1, Switch1/2
  Sum2/1 -> Relay2/1
  Relay2/1 -> Switch2/2
  Abs/1 -> Sum2/2
  Abs1/1 -> Sum1/2
  Constant2/1 -> Gain/1

== system bike_model/Maxon Motor/Velocity Saturation wrt Max and Min Handle Bar Angles ==
  Reference Velocity : Inport
  States : Inport  Port=2
  AND : Logic  IconShape=distinctive  AllPortsSameDT=off  OutDataTypeStr=boolean
  AND1 : Logic  IconShape=distinctive  AllPortsSameDT=off  OutDataTypeStr=boolean
  Compare To Constant : simulink/Logic and Bit Operations/Compare To Constant  relop=>=  const=max_handlebar  OutDataTypeStr=boolean
  Compare To Constant1 : simulink/Logic and Bit Operations/Compare To Constant  relop=<=  const=min_handlebar  OutDataTypeStr=boolean
  Compare To Zero : simulink/Logic and Bit Operations/Compare To Zero  relop=>=  OutDataTypeStr=boolean
  Compare To Zero1 : simulink/Logic and Bit Operations/Compare To Zero  relop=<=  OutDataTypeStr=boolean
  Constant : Constant  Value=0
  Demux : Demux  Outputs=3
  OR : Logic  Operator=OR  IconShape=distinctive  AllPortsSameDT=off  OutDataTypeStr=boolean
  Switch : Switch  Criteria=u2 > Threshold
  Output Velocity : Outport
  wires:
  Switch/1 -> Output Velocity/1
  Constant/1 -> Switch/1
  States/1 -> Demux/1
  Compare To Zero/1 -> AND/1
  Compare To Zero1/1 -> AND1/2
  Demux/2 -> Compare To Constant/1, Compare To Constant1/1
  Compare To Constant1/1 -> AND1/1
  AND/1 -> OR/1
  AND1/1 -> OR/2
  Compare To Constant/1 -> AND/2
  OR/1 -> Switch/2
  Reference Velocity/1 -> Compare To Zero1/1, Compare To Zero/1, Switch/3

== system bike_model/Physical Bike/A (continuous) ==
  Velocity : Inport
  1-D Lookup Table10 : Lookup_n-D  NumberOfTableDimensions=1  BreakpointsForDimension1=velocity_lqr  BreakpointsForDimension2=velocity_lqr  BreakpointsForDimension3=velocity_lqr  BreakpointsForDimension4=velocity_lqr  Table=A_full(:,1,2)  InternalRulePriority=Speed  RndMeth=Simplest  InputSameDT=on
  1-D Lookup Table11 : Lookup_n-D  NumberOfTableDimensions=1  BreakpointsForDimension1=velocity_lqr  BreakpointsForDimension2=velocity_lqr  BreakpointsForDimension3=velocity_lqr  BreakpointsForDimension4=velocity_lqr  Table=A_full(:,1,3)  InternalRulePriority=Speed  RndMeth=Simplest  InputSameDT=on
  1-D Lookup Table12 : Lookup_n-D  NumberOfTableDimensions=1  BreakpointsForDimension1=velocity_lqr  BreakpointsForDimension2=velocity_lqr  BreakpointsForDimension3=velocity_lqr  BreakpointsForDimension4=velocity_lqr  Table=A_full(:,2,1)  InternalRulePriority=Speed  RndMeth=Simplest  InputSameDT=on
  1-D Lookup Table13 : Lookup_n-D  NumberOfTableDimensions=1  BreakpointsForDimension1=velocity_lqr  BreakpointsForDimension2=velocity_lqr  BreakpointsForDimension3=velocity_lqr  BreakpointsForDimension4=velocity_lqr  Table=A_full(:,2,2)  InternalRulePriority=Speed  RndMeth=Simplest  InputSameDT=on
  1-D Lookup Table14 : Lookup_n-D  NumberOfTableDimensions=1  BreakpointsForDimension1=velocity_lqr  BreakpointsForDimension2=velocity_lqr  BreakpointsForDimension3=velocity_lqr  BreakpointsForDimension4=velocity_lqr  Table=A_full(:,2,3)  InternalRulePriority=Speed  RndMeth=Simplest  InputSameDT=on
  1-D Lookup Table15 : Lookup_n-D  NumberOfTableDimensions=1  BreakpointsForDimension1=velocity_lqr  BreakpointsForDimension2=velocity_lqr  BreakpointsForDimension3=velocity_lqr  BreakpointsForDimension4=velocity_lqr  Table=A_full(:,3,1)  InternalRulePriority=Speed  RndMeth=Simplest  InputSameDT=on
  1-D Lookup Table16 : Lookup_n-D  NumberOfTableDimensions=1  BreakpointsForDimension1=velocity_lqr  BreakpointsForDimension2=velocity_lqr  BreakpointsForDimension3=velocity_lqr  BreakpointsForDimension4=velocity_lqr  Table=A_full(:,3,2)  InternalRulePriority=Speed  RndMeth=Simplest  InputSameDT=on
  1-D Lookup Table17 : Lookup_n-D  NumberOfTableDimensions=1  BreakpointsForDimension1=velocity_lqr  BreakpointsForDimension2=velocity_lqr  BreakpointsForDimension3=velocity_lqr  BreakpointsForDimension4=velocity_lqr  Table=A_full(:,3,3)  InternalRulePriority=Speed  RndMeth=Simplest  InputSameDT=on
  1-D Lookup Table3 : Lookup_n-D  NumberOfTableDimensions=1  BreakpointsForDimension1=velocity_lqr  BreakpointsForDimension2=velocity_lqr  BreakpointsForDimension3=velocity_lqr  BreakpointsForDimension4=velocity_lqr  Table=A_full(:,1,1)  InternalRulePriority=Speed  RndMeth=Simplest  InputSameDT=on
  Display1 : Display
      settings: Decimation=9
  Matrix Concatenate3 : Concatenate  NumInputs=3  Mode=Multidimensional array  ConcatenateDimension=2
  Matrix Concatenate5 : Concatenate  NumInputs=3  Mode=Multidimensional array  ConcatenateDimension=2
  Matrix Concatenate6 : Concatenate  NumInputs=3  Mode=Multidimensional array  ConcatenateDimension=2
  Matrix Concatenate7 : Concatenate  NumInputs=3  Mode=Multidimensional array
  A : Outport
  wires:
  1-D Lookup Table13/1 -> Matrix Concatenate5/2  "A22"
  Matrix Concatenate5/1 -> Matrix Concatenate7/2
  1-D Lookup Table11/1 -> Matrix Concatenate3/3  "A13"
  Matrix Concatenate6/1 -> Matrix Concatenate7/3
  1-D Lookup Table15/1 -> Matrix Concatenate6/1  "A31"
  Velocity/1 -> 1-D Lookup Table3/1, 1-D Lookup Table10/1, 1-D Lookup Table11/1, 1-D Lookup Table12/1, 1-D Lookup Table17/1, 1-D Lookup Table16/1, 1-D Lookup Table15/1, 1-D Lookup Table14/1, 1-D Lookup Table13/1
  1-D Lookup Table14/1 -> Matrix Concatenate5/3  "A23"
  1-D Lookup Table12/1 -> Matrix Concatenate5/1  "A21"
  1-D Lookup Table3/1 -> Matrix Concatenate3/1  "A11"
  1-D Lookup Table16/1 -> Matrix Concatenate6/2  "A32"
  Matrix Concatenate3/1 -> Matrix Concatenate7/1
  1-D Lookup Table10/1 -> Matrix Concatenate3/2  "A12"
  1-D Lookup Table17/1 -> Matrix Concatenate6/3  "A33"
  Matrix Concatenate7/1 -> Display1/1, A/1

== system bike_model/Physical Bike/Accelerometer ==
  note: check the signs!
  Lateral Acceleration of the IMU due to Roll : Inport
  Centripetal Acceleration due to Path Curvature : Inport  Port=2
  True Velocity : Inport  Port=3
  True Roll Angle : Inport  Port=4
  Cos : Trigonometry  Operator=cos
  Derivative : Derivative
  Gain1 : Gain  Gain=g
  Gain2 : Gain  Gain=g
  Gain5 : Gain  Gain=g
  Multiply : Product
  Multiply1 : Product
  Mux : Mux  Inputs=3
  Scope2 : Scope
  Sin : Trigonometry
  Sum1 : Sum  Inputs=-+
  Sum6 : Sum  Inputs=-++
  Accelerations : Outport
  wires:
  Multiply/1 -> Sum6/2
  Gain1/1 -> Sum6/3  "acc_y"
  Sin/1 -> Multiply1/2, Gain1/1
  Gain5/1 -> Mux/1  "acc_x"
  Cos/1 -> Multiply/2, Gain2/1
  Gain2/1 -> Sum1/2  "acc_z"
  Lateral Acceleration of the IMU due to Roll/1 -> Sum6/1, Scope2/1
  True Roll Angle/1 -> Sin/1, Cos/1  "Real roll angle"
  True Velocity/1 -> Derivative/1
  Derivative/1 -> Gain5/1
  Centripetal Acceleration due to Path Curvature/1 -> Multiply1/1, Multiply/1
  Multiply1/1 -> Sum1/1
  Sum1/1 -> Mux/3
  Mux/1 -> Accelerations/1
  Sum6/1 -> Mux/2

== system bike_model/Physical Bike/B (continuous) ==
  Velocity : Inport
  1-D Lookup Table10 : Lookup_n-D  NumberOfTableDimensions=1  BreakpointsForDimension1=velocity_lqr  BreakpointsForDimension2=velocity_lqr  BreakpointsForDimension3=velocity_lqr  BreakpointsForDimension4=velocity_lqr  Table=B_full(:,2)  InternalRulePriority=Speed  RndMeth=Simplest  InputSameDT=on
  1-D Lookup Table11 : Lookup_n-D  NumberOfTableDimensions=1  BreakpointsForDimension1=velocity_lqr  BreakpointsForDimension2=velocity_lqr  BreakpointsForDimension3=velocity_lqr  BreakpointsForDimension4=velocity_lqr  Table=B_full(:,3)  InternalRulePriority=Speed  RndMeth=Simplest  InputSameDT=on
  1-D Lookup Table3 : Lookup_n-D  NumberOfTableDimensions=1  BreakpointsForDimension1=velocity_lqr  BreakpointsForDimension2=velocity_lqr  BreakpointsForDimension3=velocity_lqr  BreakpointsForDimension4=velocity_lqr  Table=B_full(:,1)  InternalRulePriority=Speed  RndMeth=Simplest  InputSameDT=on
  Display1 : Display
  Matrix Concatenate3 : Concatenate  NumInputs=3  Mode=Multidimensional array
  B : Outport
  wires:
  1-D Lookup Table11/1 -> Matrix Concatenate3/3  "B3"
  Velocity/1 -> 1-D Lookup Table3/1, 1-D Lookup Table11/1, 1-D Lookup Table10/1
  1-D Lookup Table3/1 -> Matrix Concatenate3/1  "B1"
  1-D Lookup Table10/1 -> Matrix Concatenate3/2  "B2"
  Matrix Concatenate3/1 -> Display1/1, B/1

== system bike_model/Physical Bike/Centripetal Acceleration Calculator ==
  True Steering Angle : Inport
  True Velocity : Inport  Port=2
  Divide : Product  Inputs=*/
  Multiply : Product
  Square : Math  Operator=square  SaturateOnIntegerOverflow=on
  Tan : Trigonometry  Operator=tan
  b : Constant  Value=b
  Centripetal Acceleration : Outport
  wires:
  True Velocity/1 -> Square/1
  Square/1 -> Divide/1
  b/1 -> Divide/2
  True Steering Angle/1 -> Tan/1
  Divide/1 -> Multiply/1
  Tan/1 -> Multiply/2
  Multiply/1 -> Centripetal Acceleration/1

== system bike_model/Physical Bike/Lateral Acceleration (due to Roll) Calculator ==
  True Roll Rate : Inport
  Constant3 : Constant  Value=IMU_height
  Derivative : Derivative
  Multiply : Product
  Scope : Scope  NumInputPorts=2
  Lateral Acceleration : Outport
  wires:
  Derivative/1 -> Scope/2, Lateral Acceleration/1
  Constant3/1 -> Multiply/1
  Multiply/1 -> Scope/1, Derivative/1
  True Roll Rate/1 -> Multiply/2

== system bike_model/Reference Position and Direction in Global CS with variable Look Ahead/Reference Position and Angle Selector ==
  total travelled distance : Inport
  1-D Lookup Table : Lookup_n-D  NumberOfTableDimensions=1  BreakpointsForDimension1=cumulative_dist_along_path  Table=path_x  ExtrapMethod=Clip  DiagnosticForOutOfRangeInput=Error  InternalRulePriority=Speed  RndMeth=Simplest  InputSameDT=on
  1-D Lookup Table1 : Lookup_n-D  NumberOfTableDimensions=1  BreakpointsForDimension1=cumulative_dist_along_path  Table=path_y  ExtrapMethod=Clip  DiagnosticForOutOfRangeInput=Error  InternalRulePriority=Speed  RndMeth=Simplest  InputSameDT=on
  Atan2 : Trigonometry  Operator=atan2
  Derivative : Derivative
  Derivative1 : Derivative
  Scope : Scope
  Unwrap : dspsigops/Unwrap  tol=pi  InputProcessing=Columns as channels (frame based)  running=off
  X_sigma : Outport
  Y_sigma : Outport  Port=2
  psi_sigma : Outport  Port=3
  wires:
  total travelled distance/1 -> 1-D Lookup Table1/1, 1-D Lookup Table/1
  Unwrap/1 -> Scope/1, psi_sigma/1
  1-D Lookup Table/1 -> X_sigma/1, Derivative1/1  "interpolated path x value"
  Derivative1/1 -> Atan2/2  "dx"
  Derivative/1 -> Atan2/1  "dy"
  Atan2/1 -> Unwrap/1
  1-D Lookup Table1/1 -> Y_sigma/1, Derivative/1  "interpolated path y value"

== system bike_model/Reference Position and Direction in Global CS with variable Look Ahead/Subsystem1 ==
  total travelled distance : Inport
  1-D Lookup Table : Lookup_n-D  NumberOfTableDimensions=1  BreakpointsForDimension1=cumulative_dist_along_path  Table=path_x  ExtrapMethod=Clip  DiagnosticForOutOfRangeInput=Error  InternalRulePriority=Speed  RndMeth=Simplest  InputSameDT=on
  1-D Lookup Table1 : Lookup_n-D  NumberOfTableDimensions=1  BreakpointsForDimension1=cumulative_dist_along_path  Table=path_y  ExtrapMethod=Clip  DiagnosticForOutOfRangeInput=Error  InternalRulePriority=Speed  RndMeth=Simplest  InputSameDT=on
  Atan2 : Trigonometry  Operator=atan2
  Derivative : Derivative
  Derivative1 : Derivative
  Scope : Scope
  Unwrap : dspsigops/Unwrap  tol=pi  InputProcessing=Columns as channels (frame based)  running=off
  X_sigma : Outport
  Y_sigma : Outport  Port=2
  psi_sigma : Outport  Port=3
  wires:
  total travelled distance/1 -> 1-D Lookup Table1/1, 1-D Lookup Table/1
  Unwrap/1 -> Scope/1, psi_sigma/1
  1-D Lookup Table/1 -> X_sigma/1, Derivative1/1  "interpolated path x value"
  Derivative1/1 -> Atan2/2  "dx"
  Derivative/1 -> Atan2/1  "dy"
  Atan2/1 -> Unwrap/1
  1-D Lookup Table1/1 -> Y_sigma/1, Derivative/1  "interpolated path y value"

== system bike_model/State Estimator/A (continuous) ==
  Velocity : Inport
  1-D Lookup Table10 : Lookup_n-D  NumberOfTableDimensions=1  BreakpointsForDimension1=velocity_lqr  BreakpointsForDimension2=velocity_lqr  BreakpointsForDimension3=velocity_lqr  BreakpointsForDimension4=velocity_lqr  Table=A_full(:,1,2)  InternalRulePriority=Speed  RndMeth=Simplest  InputSameDT=on
  1-D Lookup Table11 : Lookup_n-D  NumberOfTableDimensions=1  BreakpointsForDimension1=velocity_lqr  BreakpointsForDimension2=velocity_lqr  BreakpointsForDimension3=velocity_lqr  BreakpointsForDimension4=velocity_lqr  Table=A_full(:,1,3)  InternalRulePriority=Speed  RndMeth=Simplest  InputSameDT=on
  1-D Lookup Table12 : Lookup_n-D  NumberOfTableDimensions=1  BreakpointsForDimension1=velocity_lqr  BreakpointsForDimension2=velocity_lqr  BreakpointsForDimension3=velocity_lqr  BreakpointsForDimension4=velocity_lqr  Table=A_full(:,2,1)  InternalRulePriority=Speed  RndMeth=Simplest  InputSameDT=on
  1-D Lookup Table13 : Lookup_n-D  NumberOfTableDimensions=1  BreakpointsForDimension1=velocity_lqr  BreakpointsForDimension2=velocity_lqr  BreakpointsForDimension3=velocity_lqr  BreakpointsForDimension4=velocity_lqr  Table=A_full(:,2,2)  InternalRulePriority=Speed  RndMeth=Simplest  InputSameDT=on
  1-D Lookup Table14 : Lookup_n-D  NumberOfTableDimensions=1  BreakpointsForDimension1=velocity_lqr  BreakpointsForDimension2=velocity_lqr  BreakpointsForDimension3=velocity_lqr  BreakpointsForDimension4=velocity_lqr  Table=A_full(:,2,3)  InternalRulePriority=Speed  RndMeth=Simplest  InputSameDT=on
  1-D Lookup Table15 : Lookup_n-D  NumberOfTableDimensions=1  BreakpointsForDimension1=velocity_lqr  BreakpointsForDimension2=velocity_lqr  BreakpointsForDimension3=velocity_lqr  BreakpointsForDimension4=velocity_lqr  Table=A_full(:,3,1)  InternalRulePriority=Speed  RndMeth=Simplest  InputSameDT=on
  1-D Lookup Table16 : Lookup_n-D  NumberOfTableDimensions=1  BreakpointsForDimension1=velocity_lqr  BreakpointsForDimension2=velocity_lqr  BreakpointsForDimension3=velocity_lqr  BreakpointsForDimension4=velocity_lqr  Table=A_full(:,3,2)  InternalRulePriority=Speed  RndMeth=Simplest  InputSameDT=on
  1-D Lookup Table17 : Lookup_n-D  NumberOfTableDimensions=1  BreakpointsForDimension1=velocity_lqr  BreakpointsForDimension2=velocity_lqr  BreakpointsForDimension3=velocity_lqr  BreakpointsForDimension4=velocity_lqr  Table=A_full(:,3,3)  InternalRulePriority=Speed  RndMeth=Simplest  InputSameDT=on
  1-D Lookup Table3 : Lookup_n-D  NumberOfTableDimensions=1  BreakpointsForDimension1=velocity_lqr  BreakpointsForDimension2=velocity_lqr  BreakpointsForDimension3=velocity_lqr  BreakpointsForDimension4=velocity_lqr  Table=A_full(:,1,1)  InternalRulePriority=Speed  RndMeth=Simplest  InputSameDT=on
  Display1 : Display
      settings: Decimation=9
  Matrix Concatenate3 : Concatenate  NumInputs=3  Mode=Multidimensional array  ConcatenateDimension=2
  Matrix Concatenate5 : Concatenate  NumInputs=3  Mode=Multidimensional array  ConcatenateDimension=2
  Matrix Concatenate6 : Concatenate  NumInputs=3  Mode=Multidimensional array  ConcatenateDimension=2
  Matrix Concatenate7 : Concatenate  NumInputs=3  Mode=Multidimensional array
  A : Outport
  wires:
  1-D Lookup Table13/1 -> Matrix Concatenate5/2  "A22"
  Matrix Concatenate5/1 -> Matrix Concatenate7/2
  1-D Lookup Table11/1 -> Matrix Concatenate3/3  "A13"
  Matrix Concatenate6/1 -> Matrix Concatenate7/3
  1-D Lookup Table15/1 -> Matrix Concatenate6/1  "A31"
  Velocity/1 -> 1-D Lookup Table3/1, 1-D Lookup Table10/1, 1-D Lookup Table11/1, 1-D Lookup Table12/1, 1-D Lookup Table17/1, 1-D Lookup Table16/1, 1-D Lookup Table15/1, 1-D Lookup Table14/1, 1-D Lookup Table13/1
  1-D Lookup Table14/1 -> Matrix Concatenate5/3  "A23"
  1-D Lookup Table12/1 -> Matrix Concatenate5/1  "A21"
  1-D Lookup Table3/1 -> Matrix Concatenate3/1  "A11"
  1-D Lookup Table16/1 -> Matrix Concatenate6/2  "A32"
  Matrix Concatenate3/1 -> Matrix Concatenate7/1
  1-D Lookup Table10/1 -> Matrix Concatenate3/2  "A12"
  1-D Lookup Table17/1 -> Matrix Concatenate6/3  "A33"
  Matrix Concatenate7/1 -> Display1/1, A/1
